simulink model "ABS_brake"  (R2019b)
settings: Solver=VariableStepAuto  StartTime=0.0  StopTime=15  RelTol=1e-3
values from neighbouring files (symbols this model uses):
  ctrl = 1    [ABS_Datas.m]    (also in matlab_ABSdata.mat)
  g = 32.1800    (= 32.18)    [ABS_Datas.m]    (also in matlab_ABSdata.mat)
  I = 5    [ABS_Datas.m]    (also in matlab_ABSdata.mat)
  Kf = 1    [ABS_Datas.m]    (also in Suspension_Datas.m = 28000; matlab_ABSdata.mat; matlab_suspensiondata.mat = 28000)
  m = 50    [ABS_Datas.m]    (also in matlab_ABSdata.mat)
  PBmax = 1500    [ABS_Datas.m]    (also in matlab_ABSdata.mat)
  Rr = 1.25    [ABS_Datas.m]    (also in matlab_ABSdata.mat)
  TB = 0.01    [ABS_Datas.m]    (also in matlab_ABSdata.mat)
  v0 = 88    [ABS_Datas.m]    (also in matlab_ABSdata.mat)
settings Model: Creator=Yogesh  LastModifiedBy=Yogesh

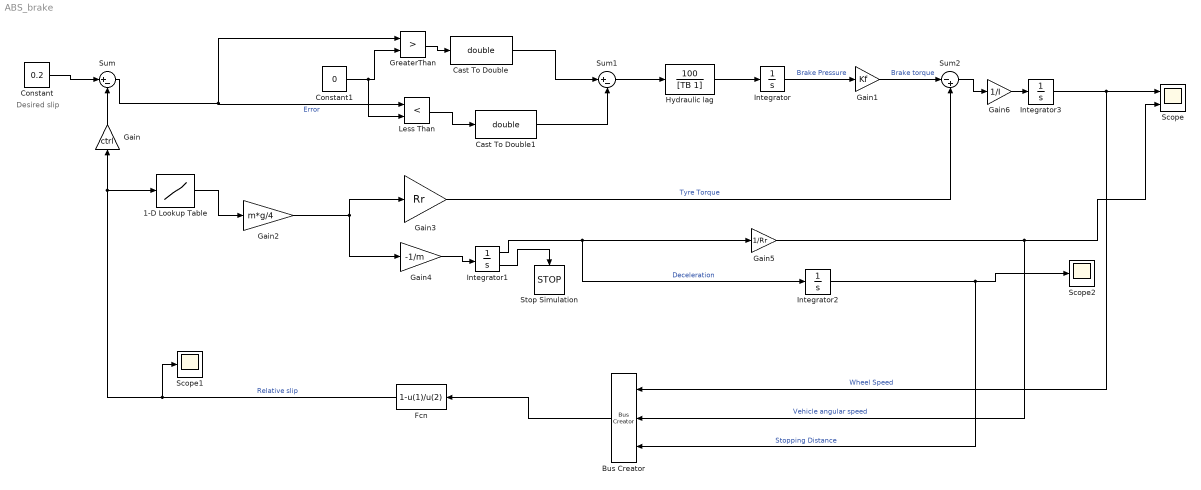
== system ABS_brake ==
  note: Desired slip
  1-D Lookup Table : Lookup_n-D  NumberOfTableDimensions=1  BreakpointsForDimension1=[0,0.05,0.1,0.15,0.2,0.25,0.3,0.35,0.4,0.45,0.5,0.55,0.6,0.65,0.70,0.75,0.80,0.85,0.90,0.95,1]  Table=[0,.4,0.8,0.97,1,0.98,0.96,0.94,0.92,0.9,0.88,0.855,0.83,0.81,0.79,0.77,0.75,0.73,0.72,0.71,0.7]  InternalRulePriority=Speed  RndMeth=Simplest  InputSameDT=on
  Bus Creator : BusCreator  Inputs=3
  Cast To Double : DataTypeConversion  OutDataTypeStr=double  RndMeth=Zero
  Cast To Double1 : DataTypeConversion  OutDataTypeStr=double  RndMeth=Zero
  Constant : Constant  Value=0.2
  Constant1 : Constant  Value=0
  Fcn : Fcn  Expr=1-u(1)/u(2)
  Gain : Gain  Gain=ctrl
  Gain1 : Gain  Gain=Kf
  Gain2 : Gain  Gain=m*g/4
  Gain3 : Gain  Gain=Rr
  Gain4 : Gain  Gain=-1/m
  Gain5 : Gain  Gain=1/Rr
  Gain6 : Gain  Gain=1/I
  GreaterThan : RelationalOperator  Operator=>  OutDataTypeStr=boolean  RndMeth=Simplest
  Hydraulic lag : TransferFcn  Numerator=[100]  Denominator=[TB 1]
  Integrator : Integrator  LimitOutput=on  UpperSaturationLimit=PBmax  LowerSaturationLimit=0
  Integrator1 : Integrator  InitialCondition=v0  LimitOutput=on  UpperSaturationLimit=1000  LowerSaturationLimit=0  ShowSaturationPort=on
  Integrator2 : Integrator
  Integrator3 : Integrator  InitialCondition=v0/Rr  LimitOutput=on  UpperSaturationLimit=1000  LowerSaturationLimit=0
  Less Than : RelationalOperator  Operator=<  OutDataTypeStr=boolean  RndMeth=Simplest
  Scope : Scope  NumInputPorts=2
  Scope1 : Scope
  Scope2 : Scope
  Stop Simulation : Stop
  Sum : Sum  Inputs=|+-
  Sum1 : Sum  Inputs=|+-
  Sum2 : Sum  Inputs=|-+
  wires:
  Gain/1 -> Sum/2
  Constant/1 -> Sum/1
  Sum/1 -> Less Than/1, GreaterThan/1  "Error"
  Constant1/1 -> Less Than/2, GreaterThan/2
  Less Than/1 -> Cast To Double1/1
  GreaterThan/1 -> Cast To Double/1
  Cast To Double/1 -> Sum1/1
  Cast To Double1/1 -> Sum1/2
  Sum1/1 -> Hydraulic lag/1
  Hydraulic lag/1 -> Integrator/1
  Gain1/1 -> Sum2/1  "Brake torque"
  Integrator/1 -> Gain1/1  "Brake Pressure"
  Gain2/1 -> Gain3/1, Gain4/1
  Gain3/1 -> Sum2/2  "Tyre Torque"
  Gain4/1 -> Integrator1/1
  Integrator1/2 -> Stop Simulation/1
  Integrator1/1 -> Integrator2/1, Gain5/1  "Deceleration"
  Gain5/1 -> Bus Creator/2, Scope/2  "Vehicle angular speed"
  Integrator2/1 -> Bus Creator/3, Scope2/1  "Stopping Distance"
  1-D Lookup Table/1 -> Gain2/1
  Sum2/1 -> Gain6/1
  Gain6/1 -> Integrator3/1
  Integrator3/1 -> Bus Creator/1, Scope/1  "Wheel Speed"
  Bus Creator/1 -> Fcn/1
  Fcn/1 -> Scope1/1, 1-D Lookup Table/1, Gain/1  "Relative slip"
